simulink model "zad2_sim"  (R2023b)
settings: Solver=VariableStepAuto  StartTime=0.0  StopTime=7  MaxStep=10e-3  RelTol=1e-3
values from neighbouring files (symbols this model uses):
  g = 9.81    [riadenieManipulatoraAplikacia.m]
  l1 = 0.25    [riadenieManipulatoraAplikacia.m]
  l2 = 0.25    [riadenieManipulatoraAplikacia.m]
  q1_zelane = 0    [riadenieManipulatoraAplikacia.m]
  q2_zelane = 0    [riadenieManipulatoraAplikacia.m]
undefined symbols (not defined in the file or in its folder): B1, B2, D1, D2, I1, I2, m1, m2, P1, P2, q1_init, q2_init, sat1low, sat1up, sat2low, sat2up
libraries: slpidlib x2
settings Model: Creator=Michal_backup  LastModifiedBy=Michal_backup

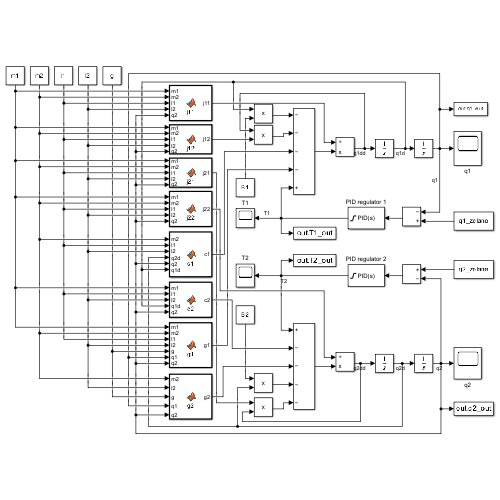
[thumbnail: Simulink's stored preview of the top-level diagram]
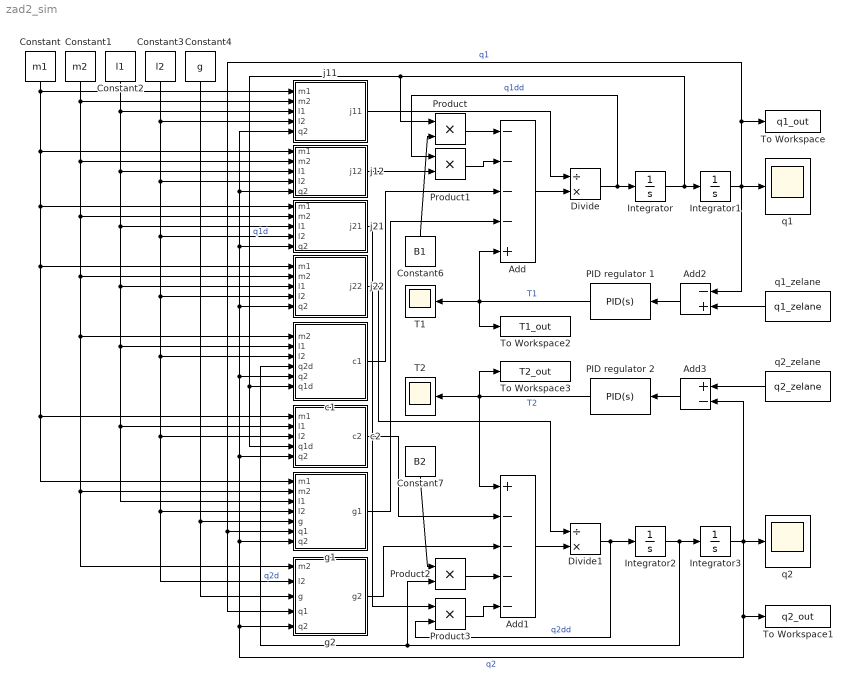
== system zad2_sim ==
  Add : Sum  Inputs=----+
  Add1 : Sum  Inputs=+----
  Add2 : Sum  Inputs=-+
  Add3 : Sum  Inputs=+-
  Constant : Constant  Value=m1
  Constant1 : Constant  Value=m2
  Constant2 : Constant  Value=l1
  Constant3 : Constant  Value=l2
  Constant4 : Constant  Value=g
  Constant6 : Constant  Value=B1
  Constant7 : Constant  Value=B2
  Divide : Product  Inputs=/*
  Divide1 : Product  Inputs=/*
  Integrator : Integrator
  Integrator1 : Integrator  InitialCondition=q1_init
  Integrator2 : Integrator
  Integrator3 : Integrator  InitialCondition=q2_init
  PID regulator 1 : slpidlib/PID Controller  Controller=PID  Form=Parallel  TimeDomain=Continuous-time  UseExternalTs=off  SampleTime=-1  IntegratorMethod=Forward Euler  FilterMethod=Forward Euler  ControllerParametersSource=internal  P=P1  I=I1  UseKiTs=off  D=D1  N=10  UseFilter=on  TunerSelectOption=Transfer Function Based (PID Tuner App)  InitialConditionSource=internal  InitialConditionForIntegrator=0  InitialConditionForFilter=0  DifferentiatorICPrevScaledInput=0  ExternalReset=none  TrackingMode=off  Kt=1  LimitOutput=on  SatLimitsSource=internal  UpperSaturationLimit=sat1up  LowerSaturationLimit=sat1low  LinearizeAsGain=on  AntiWindupMode=back-calculation  Kb=1  LimitIntegrator=on  UpperIntegratorSaturationLimit=sat1up  LowerIntegratorSaturationLimit=sat1low  POutMin=[]  POutMax=[]  IOutMin=[]  IOutMax=[]  DOutMin=[]  DOutMax=[]  NOutMin=[]  NOutMax=[]  SumOutMin=[]  SumOutMax=[]  SaturationOutMin=[]  SaturationOutMax=[]  PParamMin=[]  PParamMax=[]  IParamMin=[]  IParamMax=[]  DParamMin=[]  DParamMax=[]  NParamMin=[]  NParamMax=[]  KbParamMin=[]  KbParamMax=[]  KtParamMin=[]  KtParamMax=[]  KbOutMin=[]  KbOutMax=[]  KtOutMin=[]  KtOutMax=[]  IntegratorOutMin=[]  IntegratorOutMax=[]  FilterOutMin=[]  FilterOutMax=[]  SumI1OutMin=[]  SumI1OutMax=[]  SumI2OutMin=[]  SumI2OutMax=[]  SumI3OutMin=[]  SumI3OutMax=[]  SumI4OutMin=[]  SumI4OutMax=[]  SumDOutMin=[]  SumDOutMax=[]  DifferentiatorOutMin=[]  DifferentiatorOutMax=[]  FilterDiffOutCoefMin=[]  FilterDiffOutCoefMax=[]  ReciprocalOutMin=[]  ReciprocalOutMax=[]  SumDenOutMin=[]  SumDenOutMax=[]  SumNumOutMin=[]  SumNumOutMax=[]  DivideOutMin=[]  DivideOutMax=[]  UdiffTsProdOutMin=[]  UdiffTsProdOutMax=[]  NTsProdOutMin=[]  NTsProdOutMax=[]  UintegralTsProdOutMin=[]  UintegralTsProdOutMax=[]  UngainTsProdOutMin=[]  UngainTsProdOutMax=[]  ClampingZeroOutDataTypeStr=Inherit: Inherit via back propagation  ClampingZeroOutMin=[]  ClampingZeroOutMax=[]  FilterDenConstantOutDataTypeStr=Inherit: Inherit via back propagation  FilterDenConstantOutMin=[]  FilterDenConstantOutMax=[]  PCopyOutDataTypeStr=Inherit: Inherit via back propagation  PCopyOutMin=[]  PCopyOutMax=[]  NCopyOutDataTypeStr=Inherit: Inherit via back propagation  NCopyOutMin=[]  NCopyOutMax=[]  IntegratorContinuousStateAttributes=''  IntegratorStateMustResolveToSignalObject=off  IntegratorRTWStateStorageClass=Auto  FilterContinuousStateAttributes=''  FilterStateMustResolveToSignalObject=off  FilterRTWStateStorageClass=Auto  ParallelPVariant=InternalParameters  IdealPVariant=Disabled  IVariant=InternalParameters  DVariant=InternalParameters  IntegratorVariant=Continuous  SatVariant=Enabled  AWVariant=BackCalculation  PCopyVariant=Disabled  TRVariant=Disabled  FdbkBlocksVariant=Forward  IdealPFdbkVariant=Disabled  SatFdbkVariant=Disabled  DerivativeFilterVariant=ContFilter  NVariant=InternalParameters  NCopyVariant=Disabled  FilterICVariant=InternalICsFilter  IntegratorICVariant=InternalICs  ExternalResetVariant=Disabled  TRSumVariant=Passthrough  SumFdbkVariant=Disabled  SumVariant=Sum_PID  TsampFilterVariant=InternalTs  TsampNgainVariant=Passthrough  TsampIntegralVariant=Disabled_SignalSpec  ExternalSaturationOutDataTypeStr=Inherit: Same as second input
  PID regulator 2 : slpidlib/PID Controller  Controller=PID  Form=Parallel  TimeDomain=Continuous-time  UseExternalTs=off  SampleTime=-1  IntegratorMethod=Forward Euler  FilterMethod=Forward Euler  ControllerParametersSource=internal  P=P2  I=I2  UseKiTs=off  D=D2  N=10  UseFilter=on  TunerSelectOption=Transfer Function Based (PID Tuner App)  InitialConditionSource=internal  InitialConditionForIntegrator=0  InitialConditionForFilter=0  DifferentiatorICPrevScaledInput=0  ExternalReset=none  TrackingMode=off  Kt=1  LimitOutput=on  SatLimitsSource=internal  UpperSaturationLimit=sat2up  LowerSaturationLimit=sat2low  LinearizeAsGain=on  AntiWindupMode=back-calculation  Kb=1  LimitIntegrator=on  UpperIntegratorSaturationLimit=sat2up  LowerIntegratorSaturationLimit=sat2low  POutMin=[]  POutMax=[]  IOutMin=[]  IOutMax=[]  DOutMin=[]  DOutMax=[]  NOutMin=[]  NOutMax=[]  SumOutMin=[]  SumOutMax=[]  SaturationOutMin=[]  SaturationOutMax=[]  PParamMin=[]  PParamMax=[]  IParamMin=[]  IParamMax=[]  DParamMin=[]  DParamMax=[]  NParamMin=[]  NParamMax=[]  KbParamMin=[]  KbParamMax=[]  KtParamMin=[]  KtParamMax=[]  KbOutMin=[]  KbOutMax=[]  KtOutMin=[]  KtOutMax=[]  IntegratorOutMin=[]  IntegratorOutMax=[]  FilterOutMin=[]  FilterOutMax=[]  SumI1OutMin=[]  SumI1OutMax=[]  SumI2OutMin=[]  SumI2OutMax=[]  SumI3OutMin=[]  SumI3OutMax=[]  SumI4OutMin=[]  SumI4OutMax=[]  SumDOutMin=[]  SumDOutMax=[]  DifferentiatorOutMin=[]  DifferentiatorOutMax=[]  FilterDiffOutCoefMin=[]  FilterDiffOutCoefMax=[]  ReciprocalOutMin=[]  ReciprocalOutMax=[]  SumDenOutMin=[]  SumDenOutMax=[]  SumNumOutMin=[]  SumNumOutMax=[]  DivideOutMin=[]  DivideOutMax=[]  UdiffTsProdOutMin=[]  UdiffTsProdOutMax=[]  NTsProdOutMin=[]  NTsProdOutMax=[]  UintegralTsProdOutMin=[]  UintegralTsProdOutMax=[]  UngainTsProdOutMin=[]  UngainTsProdOutMax=[]  ClampingZeroOutDataTypeStr=Inherit: Inherit via back propagation  ClampingZeroOutMin=[]  ClampingZeroOutMax=[]  FilterDenConstantOutDataTypeStr=Inherit: Inherit via back propagation  FilterDenConstantOutMin=[]  FilterDenConstantOutMax=[]  PCopyOutDataTypeStr=Inherit: Inherit via back propagation  PCopyOutMin=[]  PCopyOutMax=[]  NCopyOutDataTypeStr=Inherit: Inherit via back propagation  NCopyOutMin=[]  NCopyOutMax=[]  IntegratorContinuousStateAttributes=''  IntegratorStateMustResolveToSignalObject=off  IntegratorRTWStateStorageClass=Auto  FilterContinuousStateAttributes=''  FilterStateMustResolveToSignalObject=off  FilterRTWStateStorageClass=Auto  ParallelPVariant=InternalParameters  IdealPVariant=Disabled  IVariant=InternalParameters  DVariant=InternalParameters  IntegratorVariant=Continuous  SatVariant=Enabled  AWVariant=BackCalculation  PCopyVariant=Disabled  TRVariant=Disabled  FdbkBlocksVariant=Forward  IdealPFdbkVariant=Disabled  SatFdbkVariant=Disabled  DerivativeFilterVariant=ContFilter  NVariant=InternalParameters  NCopyVariant=Disabled  FilterICVariant=InternalICsFilter  IntegratorICVariant=InternalICs  ExternalResetVariant=Disabled  TRSumVariant=Passthrough  SumFdbkVariant=Disabled  SumVariant=Sum_PID  TsampFilterVariant=InternalTs  TsampNgainVariant=Passthrough  TsampIntegralVariant=Disabled_SignalSpec  ExternalSaturationOutDataTypeStr=Inherit: Same as second input
  Product{,1..3} (4 alike) : Product
  T1 : Scope
  T2 : Scope
  To Workspace : ToWorkspace  VariableName=q1_out  SampleTime=-1
      settings: Save2DSignal=2-D array (concatenate along first dimension)
  To Workspace1 : ToWorkspace  VariableName=q2_out  SampleTime=-1
      settings: Save2DSignal=2-D array (concatenate along first dimension)
  To Workspace2 : ToWorkspace  VariableName=T1_out  SampleTime=-1
      settings: Save2DSignal=2-D array (concatenate along first dimension)
  To Workspace3 : ToWorkspace  VariableName=T2_out  SampleTime=-1
      settings: Save2DSignal=2-D array (concatenate along first dimension)
  c1 : MATLAB Function  TreatAsAtomicUnit=on
  c2 : MATLAB Function  TreatAsAtomicUnit=on
  g1 : MATLAB Function  TreatAsAtomicUnit=on
  g2 : MATLAB Function  TreatAsAtomicUnit=on
  j11 : MATLAB Function  TreatAsAtomicUnit=on
  j12 : MATLAB Function  TreatAsAtomicUnit=on
  j21 : MATLAB Function  TreatAsAtomicUnit=on
  j22 : MATLAB Function  TreatAsAtomicUnit=on
  q1 : Scope
  q1_zelane : Constant  Value=q1_zelane
  q2 : Scope
  q2_zelane : Constant  Value=q2_zelane
  wires:
  Constant/1 -> g1/1(m1), c2/1(m1), j22/1(m1), j21/1(m1), j12/1(m1), j11/1(m1)
  Constant1/1 -> g2/1(m2), g1/2(m2), c1/1(m2), j22/2(m2), j21/2(m2), j12/2(m2), j11/2(m2)
  Constant2/1 -> j21/3(l1), j22/3(l1), g1/3(l1), c2/2(l1), c1/2(l1), j12/3(l1), j11/3(l1)
  Constant3/1 -> g2/2(l2), g1/4(l2), c2/3(l2), c1/3(l2), j22/4(l2), j21/4(l2), j12/4(l2), j11/4(l2)
  Constant4/1 -> g2/3(g), g1/5(g)
  Add/1 -> Divide/2
  j11/1(j11) -> Divide/1
  Divide/1 -> Integrator/1, Product1/1  "q1dd"
  Integrator/1 -> Integrator1/1, Product/1, c2/4(q1d), c1/6(q1d)  "q1d"
  Integrator1/1 -> Add2/1, q1/1, To Workspace/1, g1/6(q1), g2/4(q1)  "q1"
  Constant6/1 -> Product/2
  Product/1 -> Add/1
  c1/1(c1) -> Add/3
  g1/1(g1) -> Add/4
  Product1/1 -> Add/2
  Integrator2/1 -> c1/4(q2d), Product2/2, Integrator3/1  "q2d"
  Add1/1 -> Divide1/2
  Divide1/1 -> Integrator2/1, Product3/2  "q2dd"
  j22/1(j22) -> Divide1/1
  Integrator3/1 -> To Workspace1/1, g2/5(q2), g1/7(q2), c2/5(q2), c1/5(q2), j22/5(q2), j21/5(q2), j12/5(q2), j11/5(q2), q2/1, Add3/2  "q2"
  Constant7/1 -> Product2/1
  Product2/1 -> Add1/4
  j21/1(j21) -> Product3/1
  Product3/1 -> Add1/5
  c2/1(c2) -> Add1/2
  g2/1(g2) -> Add1/3
  j12/1(j12) -> Product1/2
  q2_zelane/1 -> Add3/1
  q1_zelane/1 -> Add2/2
  PID regulator 1/1 -> Add/5, T1/1, To Workspace2/1  "T1"
  Add2/1 -> PID regulator 1/1
  Add3/1 -> PID regulator 2/1
  PID regulator 2/1 -> Add1/1, To Workspace3/1, T2/1  "T2"

== matlab function zad2_sim/j12 ==
  data: m1 input; j12 output; m2 input; l1 input; l2 input; q2 input
function j12 = j12(m1,m2,l1,l2,q2)
j12 = m2*l1*l2*cos(q2) + m2*(l2^2);
end

== matlab function zad2_sim/j11 ==
  data: m1 input; j11 output; m2 input; l1 input; l2 input; q2 input
function j11 = j11(m1,m2,l1,l2,q2)
j11 = m1*(l1^2) + m2*(l1^2) + 2*m2*l1*l2*cos(q2) + m2*(l2^2);
end

== matlab function zad2_sim/j21 ==
  data: m1 input; j21 output; m2 input; l1 input; l2 input; q2 input
function j21 = j21(m1,m2,l1,l2,q2)
j21 = m2*l1*l2*cos(q2) + m2*(l2^2);
end

== matlab function zad2_sim/j22 ==
  data: m1 input; j22 output; m2 input; l1 input; l2 input; q2 input
function j22 = j22(m1,m2,l1,l2,q2)
j22 = m2*(l2^2);
end

== matlab function zad2_sim/c1 ==
  data: m2 input; l1 input; l2 input; q2d input; c1 output; q2 input; q1d input
function c1 = c1(m2,l1,l2,q2d,q2,q1d)
c1 = m2*l1*l2*q2d*sin(q2)*(2*q1d+q2d);
end

== matlab function zad2_sim/c2 ==
  data: m1 input; l1 input; l2 input; c2 output; q1d input; q2 input
function c2 = c2(m1,l1,l2,q1d,q2)
c2 = m1*l1*l2*(q1d^2)*sin(q2);
end

== matlab function zad2_sim/g1 ==
  data: m1 input; m2 input; l1 input; l2 input; g input; q1 input; g1 output; q2 input
function g1 = g1(m1,m2,l1,l2,g,q1,q2)
g1 = m1*g*l1*cos(q1)+m2*g*(l1*cos(q1)+l2*cos(q1+q2));
end

== matlab function zad2_sim/g2 ==
  data: m2 input; l2 input; g input; q1 input; q2 input; g2 output
function g2 = g2(m2,l2,g,q1,q2)
g2 = m2*g*l2*cos(q1+q2);
end
